simulink model "testsystem2proj"  (R2019b)
settings: Solver=ode23tb  StartTime=0.0  StopTime=0.02  RelTol=1e-3  AbsTol=1e-6
values from neighbouring files (symbols this model uses):
  n = abs(fix(dif/360))    [DE_12.m]
undefined symbols (not defined in the file or in its folder): b, den, dx, flagc, m, minx, num
libraries: powerlib x43, elements x21, simulink_extras x9, powerlib_extras x1
(part 1 of 2)
settings Model: ExtModeTrigMode=oneshot  ExtModeArmWhenConnect=off  Creator=PC  LastModifiedBy=jrooaa06
settings SolverCC: AutoScaleAbsTol=off
settings DataIOCC: SaveFormat=Array  SignalLoggingSaveFormat=ModelDataLogs  ReturnWorkspaceOutputs=off
settings OptimizationCC: BlockReduction=off  BooleanDataType=off  LifeSpan=inf
settings DebuggingCC: SaveWithParameterizedLinksMsg=none  UnderspecifiedInitializationDetection=Classic  MergeDetectMultiDrivingBlocksExec=none  SignalResolutionControl=TryResolveAllWithWarning  MultiTaskDSMMsg=warning  MultiTaskCondExecSysMsg=none  SFUnexpectedBacktrackingDiag=warning  SFNoUnconditionalDefaultTransitionDiag=warning  SFExecutionAtInitializationDiag=none  ArithmeticOperatorsInVariantConditions=warning
settings HardwareCC: ProdBitPerPointer=32  ProdBitPerSizeT=32  ProdBitPerPtrDiffT=32  ProdLargestAtomicFloat=None  ProdIntDivRoundTo=Undefined  ProdEndianess=Unspecified  ProdWordSize=32  ProdHWDeviceType=32-bit Generic  TargetUnknown=on
settings ModelReferenceCC: PropagateSignalLabelsOutOfModel=off
settings SFSimCC: SimUseLocalCustomCode=off  CustomCodeUndefinedFunction=UseInterfaceOnly
settings RTWCC: RTWUseLocalCustomCode=off
settings CodeAppCC: StateflowObjectComments=on
settings GRTTargetCC: TargetLangStandard=C89/C90 (ANSI)  GeneratePreprocessorConditionals=Disable all  CombineOutputUpdateFcns=off  GRTInterface=on
settings ConfigComp: CovMetricSettings=dw  CovHtmlReporting=on  CovSaveCumulativeToWorkspaceVar=on  CovSaveSingleToWorkspaceVar=on  CovExternalEMLEnable=off
settings SimscapeCC: SimscapeNormalizeSystem=off

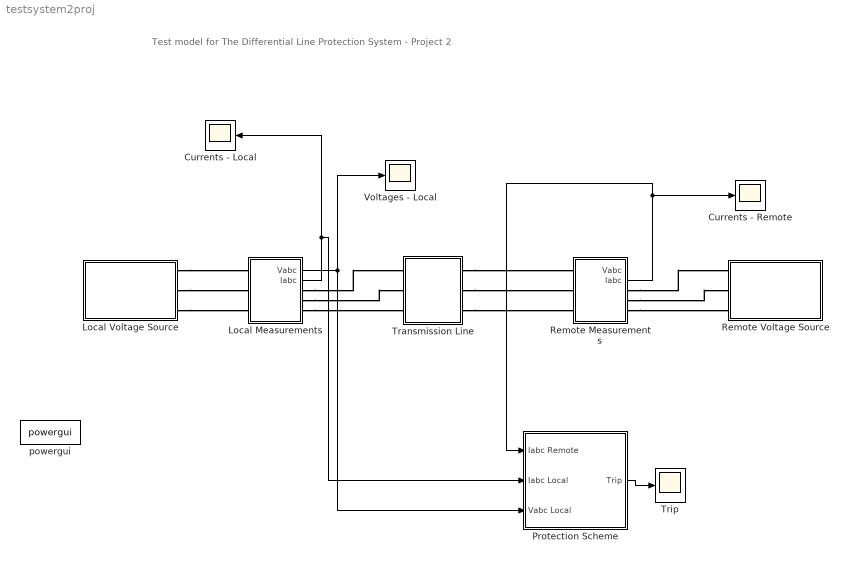
== system testsystem2proj ==
  note: Test model for The Differential Line Protection System - Project 2
  Currents - Local : Scope
  Currents - Remote : Scope
  Local Measurements : Subsystem  mask{VT=2000, CT=100}
      mask prompts: VT "VT ratio"; CT "CT ratio"
  Local Voltage Source : Subsystem  mask(3-phase inductive source - Ungrounded neutral){V=194367, Phi=10, F=60, R=3.4878, L=0.1323}
      mask prompts: V "Voltage magnitude (V) :"; Phi "Phase angle of phase A (Degrees) :"; F "Frequency (Hz) :"; R "Source resistance (Ohms):"; L "Source inductance (H) :"
      mask init:
      | a=R;b=L;c=inf;
      | short_x =[0,150];
      | short_y =[0,0];
      | 
      | resistor_x = [0 30,30,38,53,68,83,98,113,120,120,150];
      | resistor_y = [0,0,0,25,-25,25,-25,25,-25,0,0,0];
      | 
      | inductor_x = [150,173,173,174,178,184,190,197,202,205,206,204,201,201,197,196,198,201,207,214,220,225,229,229,227,224,224,220,219,221,225,230,237,243,249,252,253,251,247,247,244,243,244,248,254,260,267,272,275,276,276,300];
      | 
      | inductor_y = [0,0,1,11,19,24,25,23,17,8,-2,-12,-18,-18,-9,1,11,19,24,25,23,17,8,-2,-12,-18,-18,-9,1,11,19,24,25,23,17,8,-2,-12,-18,-18,-9,1, 11,19,24,25,23,17,8,0,0,0];
      | 
      | capacitor_x1 = [300 360 360 360];
      | capacitor_y1 = [0 0 25 -25];
      | capacitor_x2 = [390 390 390 450];
      | capacitor_y2 = [25,-25,0,0];
      | if a~=0
      | 	s1=resistor_x;
      | 	s2=resistor_y;
      | else
      | 	s1=short_x;
      | 	s2=short_y;
      | end
      | 
      | if b~=0
      | 	s3=inductor_x;
      | 	s4=inductor_y;
      | else
      | 	s3=short_x+150;
      | 	s4=short_y;
      | end
      | 
      | s5=[];
      | s6=[];
      | s7=[];
      | s8=[];
      mask Display: plot(-170,-60,360,60,s1,s2,s3,s4,s5,s6,s7,s8, [0,9,18,24,29,30,29,24,18,9,0,-9,-18,-24,-29,-30,-29,-24,-18,-9,0]*1.5-45,  [30,29,24,18,9,0,-9,-18,-24,-29,-30,-29,-24,-18,-9,0,9,18,24,29,30]*0.8,[-150,-90],[0,0],[-150,-150],[-20,20],[-165,-165],[-15,15],[-180,-180],[-10,10])
  Protection Scheme : Subsystem  mask{bias=[ 0 0;1 0.5 ;3 0.8; 5 4; 7 4.2 ; 8 4.22], Cpg=1e-6, Cpp=1e-7, zone1=[0 0 ;1 0; 1 1; 0.5 1], zone2=[0 0; 2 0; 2 2; 0 2], zone3=[0 0; 3 0; 3 3 ;0 3], zone4=[0 0; 4 0; 5 4; 1 5], reversezone=[0 0; -1 0; -1 -1; 0 -1], delay=[0.001 0.002 0.003 0.001]}
      mask prompts: bias "Bias Characteristic"; Cpg "Capacitance between phase and ground (F)"; Cpp "Mutual Capacitance between phases (F)"; zone1 "Back-up protection zone 1:"; zone2 "Back-up protection zone 2"; zone3 "Back-up protection zone 3"; zone4 "Back-up protection zone 4"; reversezone "Back-up protection reverse zone"; delay "Delay times for zone protection [Z2 Z3 Z4 Reverse]"
  Remote Measurements : Subsystem  mask{VT=2000, CT=100}
      mask prompts: VT "VT ratio"; CT "CT ratio"
  "Remote Voltage Source " : Subsystem  mask(3-phase inductive source - Ungrounded neutral){V=194367, Phi=0, F=60, R=3.4878, L=0.1323}
      mask prompts: V "Voltage magnitude (V) :"; Phi "Phase angle of phase A (Degrees) :"; F "Frequency (Hz) :"; R "Source resistance (Ohms):"; L "Source inductance (H) :"
      mask init: same as testsystem2proj/Local Voltage Source
      mask Display: plot(-170,-60,360,60,s1,s2,s3,s4,s5,s6,s7,s8, [0,9,18,24,29,30,29,24,18,9,0,-9,-18,-24,-29,-30,-29,-24,-18,-9,0]*1.5-45,  [30,29,24,18,9,0,-9,-18,-24,-29,-30,-29,-24,-18,-9,0,9,18,24,29,30]*0.8,[-150,-90],[0,0],[-150,-150],[-20,20],[-165,-165],[-15,15],[-180,-180],[-10,10])
  Transmission Line : Subsystem  mask(Teansmission line with fault){ff=60, rr=[0.0815 0.3666], ll=[2.1e-3 6.5e-3], cc=[31.6e-9 12.7e-9], length=100, faultLocation=0.5, faultType='C-A-G', faultR=0.5, faultTime=[9 10 11 12 13]}
      mask prompts: ff "Frequency used for R L C specification (Hz)"; rr "Resistance per unit length (Ohm/mile) [R1 R0]"; ll "Inductance per unit length (H/mile) [L1 L0]"; cc "Capacitance per unit length (F/mile) [C1 C0]"; length "Line length (mile)"; faultLocation "Fault location (p.u.) <0,1>"; faultType "Fault Type"; faultR "Fault Resistance per Phase (Ohm)"; faultTime "Fault time sequence (s) [C O C O C]"
      mask TypeOptions faultType: 'A-G' | 'B-G' | 'C-G' | 'B-C' | 'B-C-G' | 'C-A' | 'C-A-G' | 'A-B-C' | 'A-B-C-G'
  Trip : Scope
  Voltages - Local : Scope
  powergui : powerlib/powergui  SimulationMode=Continuous  SampleTime=1e-6  frequency=60  Iterations=50  frequencyindice=60  Pbase=100e6  ErrMax=1e-4  UnitsV=kV  UnitsW=MW  buscounter=0  FunctionMessages=off  echomessages=off  EnableUseOfTLC=off  CurrentSourceSwitches=on  DisableSnubberDevices=off  DisableRonSwitches=off  DisableVfSwitches=off  DisplayEquations=off  AutomaticDiscreteSolvers=off  SolverType=Tustin/Backward Euler (TBE)  Interpol=off  ExternalGateDelay=off  methode=off  Ts=0  x0status=blocks  SPID=off  SwTol=0  HookPort=off  NonlinearTolerance=1e-4  nMaxIteration=100  ContinueOnMaxIteration=off  RestoreLinks=warning  ResistiveCurrentMeasurement=off  Frange=[0:2:500]  Ylog=off  Xlog=on  ShowGrid=off  save=off  variable=ZData  structure=0  ZoomFFT=on  StartTime=0.0  cycles=1  DisplayStyle=1  fundamental=60  FreqAxis=off  MaxFrequency=1000  frequencyindicesteady=1  RmsSteady=1  display=off
      settings: SourceProductName=Simscape Electrical
  wires:
  Local Measurements/1(Vabc) -> Voltages - Local/1, Protection Scheme/3(Vabc Local)
  Remote Measurements/2(Iabc) -> Protection Scheme/1(Iabc Remote), Currents - Remote/1
  Protection Scheme/1(Trip) -> Trip/1
  Local Measurements/2(Iabc) -> Protection Scheme/2(Iabc Local), Currents - Local/1
  connections:
  Local Voltage Source/RConn1 -- Local Measurements/LConn1
  Local Voltage Source/RConn2 -- Local Measurements/LConn2
  Local Voltage Source/RConn3 -- Local Measurements/LConn3
  Local Measurements/RConn1 -- Transmission Line/LConn1
  Local Measurements/RConn2 -- Transmission Line/LConn2
  Local Measurements/RConn3 -- Transmission Line/LConn3
  Transmission Line/RConn1 -- Remote Measurements/LConn1
  Transmission Line/RConn2 -- Remote Measurements/LConn2
  Transmission Line/RConn3 -- Remote Measurements/LConn3
  Remote Measurements/RConn1 -- "Remote Voltage Source "/RConn1
  Remote Measurements/RConn2 -- "Remote Voltage Source "/RConn2
  Remote Measurements/RConn3 -- "Remote Voltage Source "/RConn3

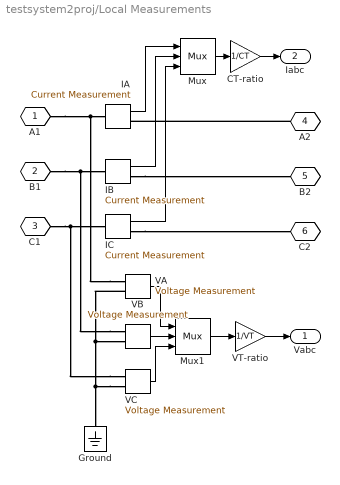
== system testsystem2proj/Local Measurements ==
  CT-ratio : Gain  Gain=1/CT  SaturateOnIntegerOverflow=on  OutDataTypeStr=Inherit: Same as input  ParamDataTypeStr=Inherit: Same as input
  Ground : powerlib/Elements/Ground  LConnTagsString=a
      settings: SourceProductName=Simscape Electrical
  IA : powerlib/Measurements/Current Measurement  PhasorSimulation=off  OutputType=Complex  PSBequivalent=0
      settings: SourceProductName=Simscape Electrical
  IB : powerlib/Measurements/Current Measurement  PhasorSimulation=off  OutputType=Complex  PSBequivalent=0
      settings: SourceProductName=Simscape Electrical
  IC : powerlib/Measurements/Current Measurement  PhasorSimulation=off  OutputType=Complex  PSBequivalent=0
      settings: SourceProductName=Simscape Electrical
  Mux : Mux  Inputs=3
  Mux1 : Mux  Inputs=3
  VA : powerlib/Measurements/Voltage Measurement  PhasorSimulation=off  OutputType=Complex  PSBequivalent=0
      settings: SourceProductName=Simscape Electrical
  VB : powerlib/Measurements/Voltage Measurement  PhasorSimulation=off  OutputType=Complex  PSBequivalent=0
      settings: SourceProductName=Simscape Electrical
  VC : powerlib/Measurements/Voltage Measurement  PhasorSimulation=off  OutputType=Complex  PSBequivalent=0
      settings: SourceProductName=Simscape Electrical
  VT-ratio : Gain  Gain=1/VT  SaturateOnIntegerOverflow=on  OutDataTypeStr=Inherit: Same as input  ParamDataTypeStr=Inherit: Same as input
  A1 : PMIOPort  Tag=PMCPort  Side=Left
  B1 : PMIOPort  Tag=PMCPort  Port=2  Side=Left
  C1 : PMIOPort  Tag=PMCPort  Port=3  Side=Left
  A2 : PMIOPort  Tag=PMCPort  Port=4  Side=Right
  B2 : PMIOPort  Tag=PMCPort  Port=5  Side=Right
  C2 : PMIOPort  Tag=PMCPort  Port=6  Side=Right
  Vabc : Outport  InitialOutput=0
  Iabc : Outport  Port=2  InitialOutput=0
  wires:
  VC/1 -> Mux1/3
  VB/1 -> Mux1/2
  VA/1 -> Mux1/1
  CT-ratio/1 -> Iabc/1
  Mux/1 -> CT-ratio/1
  VT-ratio/1 -> Vabc/1
  Mux1/1 -> VT-ratio/1
  IA/1 -> Mux/1
  IB/1 -> Mux/2
  IC/1 -> Mux/3
  connections:
  IC/RConn1 -- C2/RConn1
  IB/RConn1 -- B2/RConn1
  A2/RConn1 -- IA/RConn1
  VC/LConn1 -- IC/LConn1 -- C1/RConn1
  VB/LConn1 -- IB/LConn1 -- B1/RConn1
  VA/LConn1 -- IA/LConn1 -- A1/RConn1
  VC/LConn2 -- Ground/LConn1 -- VB/LConn2 -- VA/LConn2

== system testsystem2proj/Local Voltage Source ==
  Ground : powerlib/Elements/Ground  LConnTagsString=a
      settings: SourceProductName=Simscape Electrical
  RA : powerlib/Elements/Series RLC Branch  LConnTagsString=__new0  RConnTagsString=__new0  BranchType=RL  Resistance=R  Inductance=L  SetiL0=off  InitialCurrent=0  Capacitance=1.0  Setx0=off  InitialVoltage=0  Measurements=None
      settings: SourceProductName=Simscape Electrical
  RB : powerlib/Elements/Series RLC Branch  LConnTagsString=__new0  RConnTagsString=__new0  BranchType=RL  Resistance=R  Inductance=L  SetiL0=off  InitialCurrent=0  Capacitance=1.0  Setx0=off  InitialVoltage=0  Measurements=None
      settings: SourceProductName=Simscape Electrical
  RC : powerlib/Elements/Series RLC Branch  LConnTagsString=__new0  RConnTagsString=__new0  BranchType=RL  Resistance=R  Inductance=L  SetiL0=off  InitialCurrent=0  Capacitance=1.0  Setx0=off  InitialVoltage=0  Measurements=None
      settings: SourceProductName=Simscape Electrical
  VA : powerlib/Electrical Sources/AC Voltage Source  Amplitude=V  Phase=Phi  Frequency=F  SampleTime=0  Measurements=None  BusType=swing  Pref=10e3  Qref=0  Qmin=-inf  Qmax=+inf
      settings: SourceProductName=Simscape Electrical
  VB : powerlib/Electrical Sources/AC Voltage Source  Amplitude=V  Phase=Phi-120  Frequency=F  SampleTime=0  Measurements=None  BusType=swing  Pref=10e3  Qref=0  Qmin=-inf  Qmax=+inf
      settings: SourceProductName=Simscape Electrical
  VC : powerlib/Electrical Sources/AC Voltage Source  Amplitude=V  Phase=Phi+120  Frequency=F  SampleTime=0  Measurements=None  BusType=swing  Pref=10e3  Qref=0  Qmin=-inf  Qmax=+inf
      settings: SourceProductName=Simscape Electrical
  A : PMIOPort  Tag=PMCPort  Side=Right
  B : PMIOPort  Tag=PMCPort  Port=2  Side=Right
  C : PMIOPort  Tag=PMCPort  Port=3  Side=Right
  connections:
  VC/LConn1 -- VA/LConn1 -- Ground/LConn1 -- VB/LConn1
  VA/RConn1 -- RA/LConn1
  VB/RConn1 -- RB/LConn1
  VC/RConn1 -- RC/LConn1
  RA/RConn1 -- A/RConn1
  RB/RConn1 -- B/RConn1
  RC/RConn1 -- C/RConn1

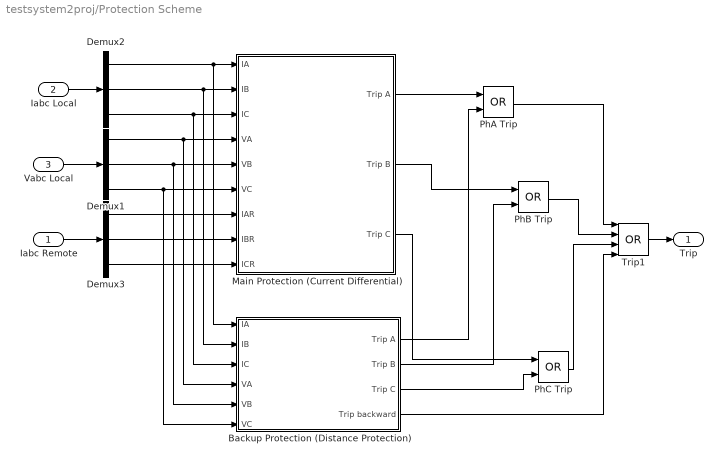
== system testsystem2proj/Protection Scheme ==
  Iabc Remote : Inport
  Iabc Local : Inport  Port=2
  Vabc Local : Inport  Port=3
  Backup Protection (Distance Protection) : Subsystem
  Demux1 : Demux  Outputs=3
  Demux2 : Demux  Outputs=3
  Demux3 : Demux  Outputs=3
  Main Protection (Current Differential) : Subsystem
  PhA Trip : Logic  Operator=OR
  PhB Trip : Logic  Operator=OR
  PhC Trip : Logic  Operator=OR
  Trip1 : Logic  Operator=OR  Inputs=4
  Trip : Outport
  wires:
  Vabc Local/1 -> Demux1/1
  Iabc Local/1 -> Demux2/1
  Iabc Remote/1 -> Demux3/1
  Trip1/1 -> Trip/1
  PhA Trip/1 -> Trip1/1
  PhB Trip/1 -> Trip1/2
  PhC Trip/1 -> Trip1/3
  Backup Protection (Distance Protection)/1(Trip A) -> PhA Trip/2
  Backup Protection (Distance Protection)/2(Trip B) -> PhB Trip/2
  Backup Protection (Distance Protection)/3(Trip C) -> PhC Trip/2
  Demux3/1 -> Main Protection (Current Differential)/7(IAR)
  Demux3/2 -> Main Protection (Current Differential)/8(IBR)
  Demux3/3 -> Main Protection (Current Differential)/9(ICR)
  Demux2/1 -> Main Protection (Current Differential)/1(IA), Backup Protection (Distance Protection)/1(IA)
  Demux2/2 -> Main Protection (Current Differential)/2(IB), Backup Protection (Distance Protection)/2(IB)
  Demux2/3 -> Main Protection (Current Differential)/3(IC), Backup Protection (Distance Protection)/3(IC)
  Demux1/1 -> Main Protection (Current Differential)/4(VA), Backup Protection (Distance Protection)/4(VA)
  Demux1/2 -> Main Protection (Current Differential)/5(VB), Backup Protection (Distance Protection)/5(VB)
  Demux1/3 -> Main Protection (Current Differential)/6(VC), Backup Protection (Distance Protection)/6(VC)
  Backup Protection (Distance Protection)/4(Trip backward) -> Trip1/4
  Main Protection (Current Differential)/1(Trip A) -> PhA Trip/1
  Main Protection (Current Differential)/2(Trip B) -> PhB Trip/1
  Main Protection (Current Differential)/3(Trip C) -> PhC Trip/1

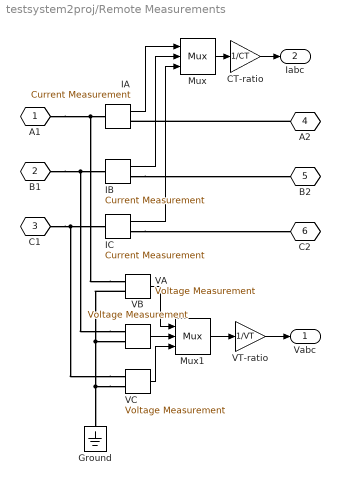
== system testsystem2proj/Remote Measurements ==
  CT-ratio : Gain  Gain=1/CT  SaturateOnIntegerOverflow=on  OutDataTypeStr=Inherit: Same as input  ParamDataTypeStr=Inherit: Same as input
  Ground : powerlib/Elements/Ground  LConnTagsString=a
      settings: SourceProductName=Simscape Electrical
  IA : powerlib/Measurements/Current Measurement  PhasorSimulation=off  OutputType=Complex  PSBequivalent=0
      settings: SourceProductName=Simscape Electrical
  IB : powerlib/Measurements/Current Measurement  PhasorSimulation=off  OutputType=Complex  PSBequivalent=0
      settings: SourceProductName=Simscape Electrical
  IC : powerlib/Measurements/Current Measurement  PhasorSimulation=off  OutputType=Complex  PSBequivalent=0
      settings: SourceProductName=Simscape Electrical
  Mux : Mux  Inputs=3
  Mux1 : Mux  Inputs=3
  VA : powerlib/Measurements/Voltage Measurement  PhasorSimulation=off  OutputType=Complex  PSBequivalent=0
      settings: SourceProductName=Simscape Electrical
  VB : powerlib/Measurements/Voltage Measurement  PhasorSimulation=off  OutputType=Complex  PSBequivalent=0
      settings: SourceProductName=Simscape Electrical
  VC : powerlib/Measurements/Voltage Measurement  PhasorSimulation=off  OutputType=Complex  PSBequivalent=0
      settings: SourceProductName=Simscape Electrical
  VT-ratio : Gain  Gain=1/VT  SaturateOnIntegerOverflow=on  OutDataTypeStr=Inherit: Same as input  ParamDataTypeStr=Inherit: Same as input
  A1 : PMIOPort  Tag=PMCPort  Side=Left
  B1 : PMIOPort  Tag=PMCPort  Port=2  Side=Left
  C1 : PMIOPort  Tag=PMCPort  Port=3  Side=Left
  A2 : PMIOPort  Tag=PMCPort  Port=4  Side=Right
  B2 : PMIOPort  Tag=PMCPort  Port=5  Side=Right
  C2 : PMIOPort  Tag=PMCPort  Port=6  Side=Right
  Vabc : Outport  InitialOutput=0
  Iabc : Outport  Port=2  InitialOutput=0
  wires:
  VC/1 -> Mux1/3
  VB/1 -> Mux1/2
  VA/1 -> Mux1/1
  CT-ratio/1 -> Iabc/1
  Mux/1 -> CT-ratio/1
  VT-ratio/1 -> Vabc/1
  Mux1/1 -> VT-ratio/1
  IA/1 -> Mux/1
  IB/1 -> Mux/2
  IC/1 -> Mux/3
  connections:
  IC/RConn1 -- C2/RConn1
  IB/RConn1 -- B2/RConn1
  A2/RConn1 -- IA/RConn1
  VC/LConn1 -- IC/LConn1 -- C1/RConn1
  VB/LConn1 -- IB/LConn1 -- B1/RConn1
  VA/LConn1 -- IA/LConn1 -- A1/RConn1
  VC/LConn2 -- Ground/LConn1 -- VB/LConn2 -- VA/LConn2

== system testsystem2proj/Remote Voltage Source  ==
  Ground : powerlib/Elements/Ground  LConnTagsString=a
      settings: SourceProductName=Simscape Electrical
  RA : powerlib/Elements/Series RLC Branch  LConnTagsString=__new0  RConnTagsString=__new0  BranchType=RL  Resistance=R  Inductance=L  SetiL0=off  InitialCurrent=0  Capacitance=1.0  Setx0=off  InitialVoltage=0  Measurements=None
      settings: SourceProductName=Simscape Electrical
  RB : powerlib/Elements/Series RLC Branch  LConnTagsString=__new0  RConnTagsString=__new0  BranchType=RL  Resistance=R  Inductance=L  SetiL0=off  InitialCurrent=0  Capacitance=1.0  Setx0=off  InitialVoltage=0  Measurements=None
      settings: SourceProductName=Simscape Electrical
  RC : powerlib/Elements/Series RLC Branch  LConnTagsString=__new0  RConnTagsString=__new0  BranchType=RL  Resistance=R  Inductance=L  SetiL0=off  InitialCurrent=0  Capacitance=1.0  Setx0=off  InitialVoltage=0  Measurements=None
      settings: SourceProductName=Simscape Electrical
  VA : powerlib/Electrical Sources/AC Voltage Source  Amplitude=V  Phase=Phi  Frequency=F  SampleTime=0  Measurements=Voltage  BusType=swing  Pref=10e3  Qref=0  Qmin=-inf  Qmax=+inf
      settings: SourceProductName=Simscape Electrical
  VB : powerlib/Electrical Sources/AC Voltage Source  Amplitude=V  Phase=Phi-120  Frequency=F  SampleTime=0  Measurements=Voltage  BusType=swing  Pref=10e3  Qref=0  Qmin=-inf  Qmax=+inf
      settings: SourceProductName=Simscape Electrical
  VC : powerlib/Electrical Sources/AC Voltage Source  Amplitude=V  Phase=Phi+120  Frequency=F  SampleTime=0  Measurements=None  BusType=swing  Pref=10e3  Qref=0  Qmin=-inf  Qmax=+inf
      settings: SourceProductName=Simscape Electrical
  A : PMIOPort  Tag=PMCPort  Side=Right
  B : PMIOPort  Tag=PMCPort  Port=2  Side=Right
  C : PMIOPort  Tag=PMCPort  Port=3  Side=Right
  connections:
  RC/RConn1 -- C/RConn1
  RB/RConn1 -- B/RConn1
  RA/RConn1 -- A/RConn1
  VC/RConn1 -- RC/LConn1
  VB/RConn1 -- RB/LConn1
  VA/RConn1 -- RA/LConn1
  VB/LConn1 -- Ground/LConn1 -- VA/LConn1 -- VC/LConn1

== system testsystem2proj/Transmission Line ==
  Fault : Subsystem
  Fault Selector : Subsystem
  Line1 : powerlib/Elements/Distributed Parameters Line  Phases=3  Frequency=ff  Resistance=rr  Inductance=ll  Capacitance=cc  Length=length*faultLocation  x1=[1.93737315649841e-10 244713.938533905 244713.938533905;376.991118430775 376.991118430775 376.991118430775;-1.14363890113431 0.490220023006083 -1.08057630378881]  x2=[4.17528404371218e-10 247270.406287336 247270.406287336;376.991118430775 376.991118430775 376.991118430775;-0.895009460576135 0.449233113533289 -1.12156321326161]  x3=[2.62101290427986e-12 709.319312320514 709.319312320518;376.991118430775 376.991118430775 376.991118430775;-2.01300464495126 0.267353068449138 -1.30344325834575]  x4=[1.05439609711696e-12 1190.69642129133 1190.69642129132;376.991118430775 376.991118430775 376.991118430775;0.959692276161214 0.466990655381244 -1.10380567141365]  x5=0.000454285152739994  V1=[1.937e-10 2.447e+05 2.447e+05;377 377 377;-1.144 0.4902 -1.081]  V2=[4.175e-10 2.473e+05 2.473e+05;377 377 377;-0.895 0.4492 -1.122]  I1=[2.621e-12 709.3 709.3;377 377 377;-2.013 0.2674 -1.303]  I2=[1.054e-12 1191 1191;377 377 377;0.9597 0.467 -1.104]  nHarmo=1  Measurements=None
      settings: SourceProductName=Simscape Electrical
  Line2 : powerlib/Elements/Distributed Parameters Line  Phases=3  Frequency=ff  Resistance=rr  Inductance=ll  Capacitance=cc  Length=length*(1-faultLocation)  x1=[4.17528404371218e-10 247270.406287336 247270.406287336;376.991118430775 376.991118430775 376.991118430775;-0.895009460576135 0.449233113533289 -1.12156321326161]  x2=[2.82547085064981e-10 244460.357066528 244460.357066528;376.991118430775 376.991118430775 376.991118430775;-0.77354881395291 0.41468188233202 -1.15611444446288]  x3=[6.1795565465611e-13 730.365390861983 730.365390861978;376.991118430775 376.991118430775 376.991118430775;-0.860185856032807 0.42028091422424 -1.15051541257066]  x4=[1.68453032078769e-12 1162.47547836006 1162.47547836006;376.991118430775 376.991118430775 376.991118430775;-2.26533611674482 0.313964295998751 -1.25683203079614]  x5=0.000454285152739994  V1=[4.175e-10 2.473e+05 2.473e+05;377 377 377;-0.895 0.4492 -1.122]  V2=[2.825e-10 2.445e+05 2.445e+05;377 377 377;-0.7735 0.4147 -1.156]  I1=[6.18e-13 730.4 730.4;377 377 377;-0.8602 0.4203 -1.151]  I2=[1.685e-12 1162 1162;377 377 377;-2.265 0.314 -1.257]  nHarmo=1  Measurements=None
      settings: SourceProductName=Simscape Electrical
  Timer : powerlib_extras/Control  Blocks/Timer  t=[0 faultTime]  e=[0 1 0 1 0 1]
      settings: SourceProductName=Simscape Electrical  SourceProductBaseCode=PS
  A1 : PMIOPort  Tag=PMCPort  Side=Left
  B1 : PMIOPort  Tag=PMCPort  Port=2  Side=Left
  C1 : PMIOPort  Tag=PMCPort  Port=3  Side=Left
  A2 : PMIOPort  Tag=PMCPort  Port=4  Side=Right
  B2 : PMIOPort  Tag=PMCPort  Port=5  Side=Right
  C2 : PMIOPort  Tag=PMCPort  Port=6  Side=Right
  wires:
  Timer/1 -> Fault/5(Tfault)
  Fault Selector/4(faultG) -> Fault/4(faultG)
  Fault Selector/3(faultC) -> Fault/3(faultC)
  Fault Selector/2(faultB) -> Fault/2(faultB)
  Fault Selector/1(faultA) -> Fault/1(faultA)
  connections:
  Line2/RConn3 -- C2/RConn1
  Line2/RConn2 -- B2/RConn1
  Line2/RConn1 -- A2/RConn1
  C1/RConn1 -- Line1/LConn3
  B1/RConn1 -- Line1/LConn2
  A1/RConn1 -- Line1/LConn1
  Fault/LConn3 -- Line1/RConn3 -- Line2/LConn3
  Fault/LConn2 -- Line2/LConn2 -- Line1/RConn2
  Fault/LConn1 -- Line2/LConn1 -- Line1/RConn1

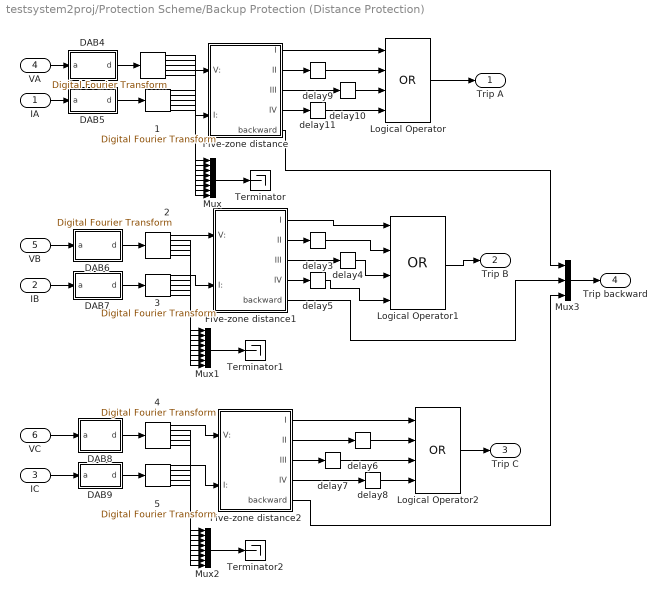
== system testsystem2proj/Protection Scheme/Backup Protection (Distance Protection) ==
  IA : Inport
  IB : Inport  Port=2
  IC : Inport  Port=3
  VA : Inport  Port=4
  VB : Inport  Port=5
  VC : Inport  Port=6
   {,1..5} (6 alike) : elements/   fo=60  window_size=40  harmonic=[1 2 3 4 5]
  DAB4 : Subsystem  mask(Data Adquisition Board){filter=off, approx=Bessel, order=2, numerator=[], denominator=[], freq=180, resdis=off, vertres=12, xmax=10, winsize=40, G=1.0, fs=60*40}
      mask prompts: filter "Disable Analog Filter"; approx "Filter approximation"; numerator "Free expression filter: numerator(descending order of s)"; denominator "Free expression filter: denominator:"; freq "Cut-off frequency"; resdis "Disable Vertical Resolution"; vertres "Vertical Resolution: No. of bits"; xmax "Vertical Resolution: signal range"; winsize "Window size"; G "Gain"; fs "Sampling frequency"
      mask help: Performs analog filtering, signal conditioning and sampling. A single signal is the input, a buffer with the signal samples is the output. The options include analog filter enable/disable switch, type, order and cut-off frequency of the analog filter, conditioning gain, sampling frequency, number of bits, the length of the buffer.
      mask init:
      | dab1
      mask TypeOptions approx: Bessel | Tschebyscheff | Butterworth | free expression
      mask TypeOptions order: 2 | 3 | 4
      mask TypeOptions vertres: 8 | 12 | 16
      mask Display: disp('DAB')
  DAB5 : Subsystem  mask(Data Adquisition Board){filter=off, approx=Bessel, order=2, numerator=[], denominator=[], freq=180, resdis=off, vertres=12, xmax=10, winsize=40, G=1.0, fs=60*40}
      mask prompts: filter "Disable Analog Filter"; approx "Filter approximation"; numerator "Free expression filter: numerator(descending order of s)"; denominator "Free expression filter: denominator:"; freq "Cut-off frequency"; resdis "Disable Vertical Resolution"; vertres "Vertical Resolution: No. of bits"; xmax "Vertical Resolution: signal range"; winsize "Window size"; G "Gain"; fs "Sampling frequency"
      mask help: Performs analog filtering, signal conditioning and sampling. A single signal is the input, a buffer with the signal samples is the output. The options include analog filter enable/disable switch, type, order and cut-off frequency of the analog filter, conditioning gain, sampling frequency, number of bits, the length of the buffer.
      mask init:
      | dab1
      mask TypeOptions approx: Bessel | Tschebyscheff | Butterworth | free expression
      mask TypeOptions order: 2 | 3 | 4
      mask TypeOptions vertres: 8 | 12 | 16
      mask Display: disp('DAB')
  DAB6 : Subsystem  mask(Data Adquisition Board){filter=off, approx=Bessel, order=2, numerator=[], denominator=[], freq=180, resdis=off, vertres=12, xmax=10, winsize=40, G=1.0, fs=60*40}
      mask prompts: filter "Disable Analog Filter"; approx "Filter approximation"; numerator "Free expression filter: numerator(descending order of s)"; denominator "Free expression filter: denominator:"; freq "Cut-off frequency"; resdis "Disable Vertical Resolution"; vertres "Vertical Resolution: No. of bits"; xmax "Vertical Resolution: signal range"; winsize "Window size"; G "Gain"; fs "Sampling frequency"
      mask help: Performs analog filtering, signal conditioning and sampling. A single signal is the input, a buffer with the signal samples is the output. The options include analog filter enable/disable switch, type, order and cut-off frequency of the analog filter, conditioning gain, sampling frequency, number of bits, the length of the buffer.
      mask init:
      | dab1
      mask TypeOptions approx: Bessel | Tschebyscheff | Butterworth | free expression
      mask TypeOptions order: 2 | 3 | 4
      mask TypeOptions vertres: 8 | 12 | 16
      mask Display: disp('DAB')
  DAB7 : Subsystem  mask(Data Adquisition Board){filter=off, approx=Bessel, order=2, numerator=[], denominator=[], freq=180, resdis=off, vertres=12, xmax=10, winsize=40, G=1.0, fs=60*40}
      mask prompts: filter "Disable Analog Filter"; approx "Filter approximation"; numerator "Free expression filter: numerator(descending order of s)"; denominator "Free expression filter: denominator:"; freq "Cut-off frequency"; resdis "Disable Vertical Resolution"; vertres "Vertical Resolution: No. of bits"; xmax "Vertical Resolution: signal range"; winsize "Window size"; G "Gain"; fs "Sampling frequency"
      mask help: Performs analog filtering, signal conditioning and sampling. A single signal is the input, a buffer with the signal samples is the output. The options include analog filter enable/disable switch, type, order and cut-off frequency of the analog filter, conditioning gain, sampling frequency, number of bits, the length of the buffer.
      mask init:
      | dab1
      mask TypeOptions approx: Bessel | Tschebyscheff | Butterworth | free expression
      mask TypeOptions order: 2 | 3 | 4
      mask TypeOptions vertres: 8 | 12 | 16
      mask Display: disp('DAB')
  DAB8 : Subsystem  mask(Data Adquisition Board){filter=off, approx=Bessel, order=2, numerator=[], denominator=[], freq=180, resdis=off, vertres=12, xmax=10, winsize=40, G=1.0, fs=60*40}
      mask prompts: filter "Disable Analog Filter"; approx "Filter approximation"; numerator "Free expression filter: numerator(descending order of s)"; denominator "Free expression filter: denominator:"; freq "Cut-off frequency"; resdis "Disable Vertical Resolution"; vertres "Vertical Resolution: No. of bits"; xmax "Vertical Resolution: signal range"; winsize "Window size"; G "Gain"; fs "Sampling frequency"
      mask help: Performs analog filtering, signal conditioning and sampling. A single signal is the input, a buffer with the signal samples is the output. The options include analog filter enable/disable switch, type, order and cut-off frequency of the analog filter, conditioning gain, sampling frequency, number of bits, the length of the buffer.
      mask init:
      | dab1
      mask TypeOptions approx: Bessel | Tschebyscheff | Butterworth | free expression
      mask TypeOptions order: 2 | 3 | 4
      mask TypeOptions vertres: 8 | 12 | 16
      mask Display: disp('DAB')
  DAB9 : Subsystem  mask(Data Adquisition Board){filter=off, approx=Bessel, order=2, numerator=[], denominator=[], freq=180, resdis=off, vertres=12, xmax=10, winsize=40, G=1.0, fs=60*40}
      mask prompts: filter "Disable Analog Filter"; approx "Filter approximation"; numerator "Free expression filter: numerator(descending order of s)"; denominator "Free expression filter: denominator:"; freq "Cut-off frequency"; resdis "Disable Vertical Resolution"; vertres "Vertical Resolution: No. of bits"; xmax "Vertical Resolution: signal range"; winsize "Window size"; G "Gain"; fs "Sampling frequency"
      mask help: Performs analog filtering, signal conditioning and sampling. A single signal is the input, a buffer with the signal samples is the output. The options include analog filter enable/disable switch, type, order and cut-off frequency of the analog filter, conditioning gain, sampling frequency, number of bits, the length of the buffer.
      mask init:
      | dab1
      mask TypeOptions approx: Bessel | Tschebyscheff | Butterworth | free expression
      mask TypeOptions order: 2 | 3 | 4
      mask TypeOptions vertres: 8 | 12 | 16
      mask Display: disp('DAB')
  Five-zone distance : Subsystem
  Five-zone distance1 : Subsystem
  Five-zone distance2 : Subsystem
  Logical Operator : Logic  Operator=OR  Inputs=4
  Logical Operator1 : Logic  Operator=OR  Inputs=4
  Logical Operator2 : Logic  Operator=OR  Inputs=4
  Mux : Mux  Inputs=8
  Mux1 : Mux  Inputs=8
  Mux2 : Mux  Inputs=8
  Mux3 : Mux  Inputs=3
  Terminator : Terminator
  Terminator1 : Terminator
  Terminator2 : Terminator
  delay10 : TransportDelay  DelayTime=delay(2)
  delay11 : TransportDelay  DelayTime=delay(3)
  delay3 : TransportDelay  DelayTime=delay(1)
  delay4 : TransportDelay  DelayTime=delay(2)
  delay5 : TransportDelay  DelayTime=delay(3)
  delay6 : TransportDelay  DelayTime=delay(1)
  delay7 : TransportDelay  DelayTime=delay(2)
  delay8 : TransportDelay  DelayTime=delay(3)
  delay9 : TransportDelay  DelayTime=delay(1)
  Trip A : Outport
  Trip B : Outport  Port=2
  Trip C : Outport  Port=3
  Trip backward : Outport  Port=4
  wires:
  Five-zone distance1/1(I) -> Logical Operator1/1
  " 4"/1 -> Five-zone distance2/1(V:)
  DAB9/1(d) -> " 5"/1
  DAB8/1(d) -> " 4"/1
  VC/1 -> DAB8/1(a)
  IC/1 -> DAB9/1(a)
  Logical Operator2/1 -> Trip C/1
  " 2"/1 -> Five-zone distance1/1(V:)
  DAB7/1(d) -> " 3"/1
  DAB6/1(d) -> " 2"/1
  " 3"/1 -> Five-zone distance1/2(I:)
  Five-zone distance1/2(II) -> delay3/1
  Five-zone distance1/3(III) -> delay4/1
  Five-zone distance1/4(IV) -> delay5/1
  delay3/1 -> Logical Operator1/2
  delay4/1 -> Logical Operator1/3
  delay5/1 -> Logical Operator1/4
  VB/1 -> DAB6/1(a)
  IB/1 -> DAB7/1(a)
  Logical Operator1/1 -> Trip B/1
  " "/1 -> Five-zone distance/1(V:)
  DAB5/1(d) -> " 1"/1
  DAB4/1(d) -> " "/1
  " 1"/1 -> Five-zone distance/2(I:)
  Five-zone distance/1(I) -> Logical Operator/1
  VA/1 -> DAB4/1(a)
  IA/1 -> DAB5/1(a)
  Logical Operator/1 -> Trip A/1
  " "/3 -> Mux/1
  " "/2 -> Mux/2
  " "/4 -> Mux/3
  " "/5 -> Mux/4
  " 1"/2 -> Mux/5
  " 1"/3 -> Mux/6
  " 1"/4 -> Mux/7
  " 1"/5 -> Mux/8
  " 2"/2 -> Mux1/1
  " 2"/3 -> Mux1/2
  " 2"/4 -> Mux1/3
  " 2"/5 -> Mux1/4
  " 3"/2 -> Mux1/5
  " 3"/3 -> Mux1/6
  " 3"/4 -> Mux1/7
  " 3"/5 -> Mux1/8
  " 4"/3 -> Mux2/1
  " 4"/2 -> Mux2/2
  " 4"/4 -> Mux2/3
  " 4"/5 -> Mux2/4
  " 5"/2 -> Mux2/5
  " 5"/3 -> Mux2/6
  " 5"/4 -> Mux2/7
  " 5"/5 -> Mux2/8
  Five-zone distance/5(backward) -> Mux3/1
  Five-zone distance1/5(backward) -> Mux3/2
  " 5"/1 -> Five-zone distance2/2(I:)
  delay6/1 -> Logical Operator2/2
  delay7/1 -> Logical Operator2/3
  delay8/1 -> Logical Operator2/4
  Five-zone distance2/1(I) -> Logical Operator2/1
  Five-zone distance2/2(II) -> delay6/1
  Five-zone distance2/3(III) -> delay7/1
  Five-zone distance2/4(IV) -> delay8/1
  Five-zone distance2/5(backward) -> Mux3/3
  Five-zone distance/2(II) -> delay9/1
  delay9/1 -> Logical Operator/2
  Five-zone distance/3(III) -> delay10/1
  Five-zone distance/4(IV) -> delay11/1
  Mux/1 -> Terminator/1
  Mux1/1 -> Terminator1/1
  Mux2/1 -> Terminator2/1
  delay10/1 -> Logical Operator/3
  delay11/1 -> Logical Operator/4
  Mux3/1 -> Trip backward/1

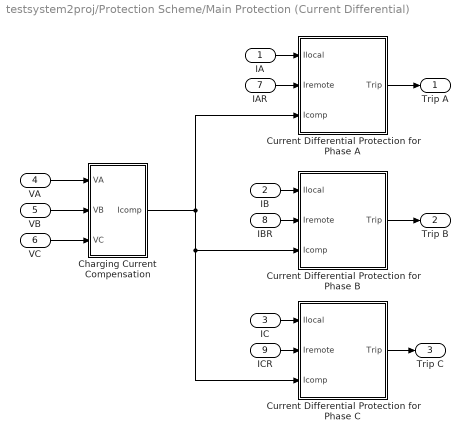
== system testsystem2proj/Protection Scheme/Main Protection (Current Differential) ==
  IA : Inport
  IB : Inport  Port=2
  IC : Inport  Port=3
  VA : Inport  Port=4
  VB : Inport  Port=5
  VC : Inport  Port=6
  IAR : Inport  Port=7
  IBR : Inport  Port=8
  ICR : Inport  Port=9
  Charging Current Compensation : Subsystem
  Current Differential Protection for Phase A : Subsystem
  Current Differential Protection for Phase B : Subsystem
  Current Differential Protection for Phase C : Subsystem
  Trip A : Outport  InitialOutput=0
  Trip B : Outport  Port=2  InitialOutput=0
  Trip C : Outport  Port=3  InitialOutput=0
  wires:
  IA/1 -> Current Differential Protection for Phase A/1(Ilocal)
  IAR/1 -> Current Differential Protection for Phase A/2(Iremote)
  IB/1 -> Current Differential Protection for Phase B/1(Ilocal)
  Current Differential Protection for Phase C/1(Trip) -> Trip C/1
  Current Differential Protection for Phase A/1(Trip) -> Trip A/1
  Current Differential Protection for Phase B/1(Trip) -> Trip B/1
  VB/1 -> Charging Current Compensation/2(VB)
  IBR/1 -> Current Differential Protection for Phase B/2(Iremote)
  IC/1 -> Current Differential Protection for Phase C/1(Ilocal)
  VA/1 -> Charging Current Compensation/1(VA)
  VC/1 -> Charging Current Compensation/3(VC)
  ICR/1 -> Current Differential Protection for Phase C/2(Iremote)
  Charging Current Compensation/1(Icomp) -> Current Differential Protection for Phase A/3(Icomp), Current Differential Protection for Phase B/3(Icomp), Current Differential Protection for Phase C/3(Icomp)

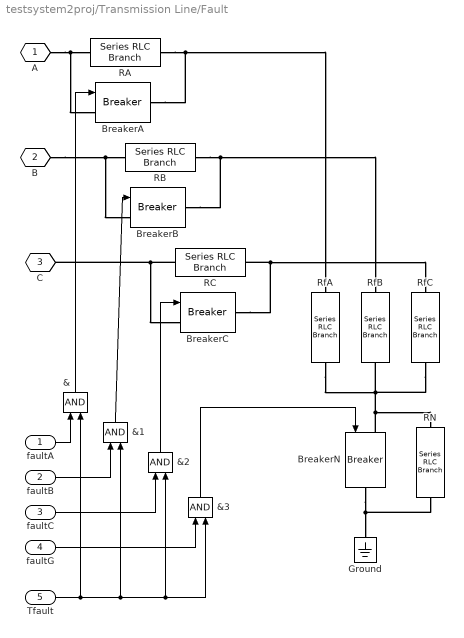
== system testsystem2proj/Transmission Line/Fault ==
  faultA : Inport
  faultB : Inport  Port=2
  faultC : Inport  Port=3
  faultG : Inport  Port=4
  Tfault : Inport  Port=5
  &{,1..3} (4 alike) : Logic
  BreakerA : powerlib/Elements/Breaker  InitialState=0  SwitchingTimes="[ 1/60  5/60 ]"  External=on  BreakerResistance=0.01  SnubberResistance=1e6  SnubberCapacitance=inf  Measurements=None  MoreParameters=off  NoBreakLoop=off
      settings: SourceProductName=Simscape Electrical
  BreakerB : powerlib/Elements/Breaker  InitialState=0  SwitchingTimes="[ 1/60  5/60 ]"  External=on  BreakerResistance=0.01  SnubberResistance=1e6  SnubberCapacitance=inf  Measurements=None  MoreParameters=off  NoBreakLoop=off
      settings: SourceProductName=Simscape Electrical
  BreakerC : powerlib/Elements/Breaker  InitialState=0  SwitchingTimes="[ 1/60  5/60 ]"  External=on  BreakerResistance=0.01  SnubberResistance=1e6  SnubberCapacitance=inf  Measurements=None  MoreParameters=off  NoBreakLoop=off
      settings: SourceProductName=Simscape Electrical
  BreakerN : powerlib/Elements/Breaker  InitialState=0  SwitchingTimes="[ 1/60  5/60 ]"  External=on  BreakerResistance=0.01  SnubberResistance=1e6  SnubberCapacitance=inf  Measurements=None  MoreParameters=off  NoBreakLoop=off
      settings: SourceProductName=Simscape Electrical
  Ground : powerlib/Elements/Ground  LConnTagsString=a
      settings: SourceProductName=Simscape Electrical
  RA : powerlib/Elements/Series RLC Branch  LConnTagsString=__new0  RConnTagsString=__new0  BranchType=R  Resistance=10000  Inductance=1e-3  SetiL0=off  InitialCurrent=0  Capacitance=1e-6  Setx0=off  InitialVoltage=0  Measurements=None
      settings: SourceProductName=Simscape Electrical
  RB : powerlib/Elements/Series RLC Branch  LConnTagsString=__new0  RConnTagsString=__new0  BranchType=R  Resistance=10000  Inductance=1e-3  SetiL0=off  InitialCurrent=0  Capacitance=1e-6  Setx0=off  InitialVoltage=0  Measurements=None
      settings: SourceProductName=Simscape Electrical
  RC : powerlib/Elements/Series RLC Branch  LConnTagsString=__new0  RConnTagsString=__new0  BranchType=R  Resistance=10000  Inductance=1e-3  SetiL0=off  InitialCurrent=0  Capacitance=1e-6  Setx0=off  InitialVoltage=0  Measurements=None
      settings: SourceProductName=Simscape Electrical
  RN : powerlib/Elements/Series RLC Branch  LConnTagsString=__new0  RConnTagsString=__new0  BranchType=R  Resistance=10000  Inductance=1e-3  SetiL0=off  InitialCurrent=0  Capacitance=1e-6  Setx0=off  InitialVoltage=0  Measurements=None
      settings: SourceProductName=Simscape Electrical
  RfA : powerlib/Elements/Series RLC Branch  LConnTagsString=__new0  RConnTagsString=__new0  BranchType=R  Resistance=faultR  Inductance=1e-3  SetiL0=off  InitialCurrent=0  Capacitance=1e-6  Setx0=off  InitialVoltage=0  Measurements=None
      settings: SourceProductName=Simscape Electrical
  RfB : powerlib/Elements/Series RLC Branch  LConnTagsString=__new0  RConnTagsString=__new0  BranchType=R  Resistance=faultR  Inductance=1e-3  SetiL0=off  InitialCurrent=0  Capacitance=1e-6  Setx0=off  InitialVoltage=0  Measurements=None
      settings: SourceProductName=Simscape Electrical
  RfC : powerlib/Elements/Series RLC Branch  LConnTagsString=__new0  RConnTagsString=__new0  BranchType=R  Resistance=faultR  Inductance=1e-3  SetiL0=off  InitialCurrent=0  Capacitance=1e-6  Setx0=off  InitialVoltage=0  Measurements=None
      settings: SourceProductName=Simscape Electrical
  A : PMIOPort  Tag=PMCPort  Side=Left
  B : PMIOPort  Tag=PMCPort  Port=2  Side=Left
  C : PMIOPort  Tag=PMCPort  Port=3  Side=Left
  wires:
  faultA/1 -> &/1
  faultB/1 -> &1/1
  faultC/1 -> &2/1
  faultG/1 -> &3/1
  Tfault/1 -> &3/2, &2/2, &1/2, &/2
  &3/1 -> BreakerN/1
  &/1 -> BreakerA/1
  &1/1 -> BreakerB/1
  &2/1 -> BreakerC/1
  connections:
  B/RConn1 -- RB/LConn1 -- BreakerB/LConn1
  A/RConn1 -- BreakerA/LConn1 -- RA/LConn1
  RC/LConn1 -- C/RConn1 -- BreakerC/LConn1
  BreakerC/RConn1 -- RC/RConn1 -- RfC/LConn1
  RB/RConn1 -- RfB/LConn1 -- BreakerB/RConn1
  RA/RConn1 -- RfA/LConn1 -- BreakerA/RConn1
  BreakerN/LConn1 -- RN/LConn1 -- RfB/RConn1 -- RfA/RConn1 -- RfC/RConn1
  BreakerN/RConn1 -- Ground/LConn1 -- RN/RConn1

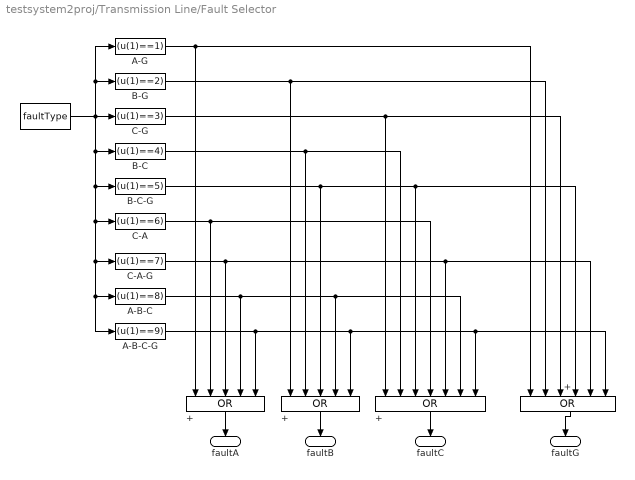
== system testsystem2proj/Transmission Line/Fault Selector ==
  " " : Constant  Value=faultType
  "  +" : Logic  Operator=OR  Inputs=7
  " +" : Logic  Operator=OR  Inputs=5
  + : Logic  Operator=OR  Inputs=5
  "+ " : Logic  Operator=OR  Inputs=6
  A-B-C : Fcn  Expr=(u(1)==8)
  A-B-C-G : Fcn  Expr=(u(1)==9)
  A-G : Fcn  Expr=(u(1)==1)
  B-C : Fcn  Expr=(u(1)==4)
  B-C-G : Fcn  Expr=(u(1)==5)
  B-G : Fcn  Expr=(u(1)==2)
  C-A : Fcn  Expr=(u(1)==6)
  C-A-G : Fcn  Expr=(u(1)==7)
  C-G : Fcn  Expr=(u(1)==3)
  faultA : Outport  InitialOutput=0
  faultB : Outport  Port=2  InitialOutput=0
  faultC : Outport  Port=3  InitialOutput=0
  faultG : Outport  Port=4  InitialOutput=0
  wires:
  " "/1 -> C-G/1, A-G/1, B-G/1, B-C/1, C-A/1, C-A-G/1, A-B-C/1, A-B-C-G/1, B-C-G/1
  +/1 -> faultA/1
  " +"/1 -> faultB/1
  "  +"/1 -> faultC/1
  "+ "/1 -> faultG/1
  A-G/1 -> "+ "/1, +/1
  C-A/1 -> "  +"/4, +/2
  B-G/1 -> " +"/1, "+ "/2
  B-C/1 -> "  +"/2, " +"/2
  B-C-G/1 -> "  +"/3, "+ "/4, " +"/3
  C-G/1 -> "  +"/1, "+ "/3
  C-A-G/1 -> "  +"/5, "+ "/5, +/3
  A-B-C-G/1 -> " +"/5, "  +"/7, "+ "/6, +/5
  A-B-C/1 -> " +"/4, "  +"/6, +/4

== system testsystem2proj/Protection Scheme/Backup Protection (Distance Protection)/DAB4 ==
  a : Inport
  AD & Buffer : S-Function  FunctionName=dab2  Parameters=winsize,fs,dx,resdis  SFunctionDeploymentMode=off  EnableBusSupport=off
  Analog Filter : TransferFcn  Numerator=num  Denominator=den
  Gain : Gain  Gain=G  SaturateOnIntegerOverflow=on  OutDataTypeStr=Inherit: Same as input  ParamDataTypeStr=Inherit: Same as input
  Zero-Order Hold : ZeroOrderHold  SampleTime=1/fs
  d : Outport  InitialOutput=[zeros(winsize,1)]
  wires:
  Analog Filter/1 -> Gain/1
  Gain/1 -> Zero-Order Hold/1
  Zero-Order Hold/1 -> AD & Buffer/1
  a/1 -> Analog Filter/1
  AD & Buffer/1 -> d/1

== system testsystem2proj/Protection Scheme/Backup Protection (Distance Protection)/DAB5 ==
  a : Inport
  AD & Buffer : S-Function  FunctionName=dab2  Parameters=winsize,fs,dx,resdis  SFunctionDeploymentMode=off  EnableBusSupport=off
  Analog Filter : TransferFcn  Numerator=num  Denominator=den
  Gain : Gain  Gain=G  SaturateOnIntegerOverflow=on  OutDataTypeStr=Inherit: Same as input  ParamDataTypeStr=Inherit: Same as input
  Zero-Order Hold : ZeroOrderHold  SampleTime=1/fs
  d : Outport  InitialOutput=[zeros(winsize,1)]
  wires:
  AD & Buffer/1 -> d/1
  a/1 -> Analog Filter/1
  Zero-Order Hold/1 -> AD & Buffer/1
  Gain/1 -> Zero-Order Hold/1
  Analog Filter/1 -> Gain/1

== system testsystem2proj/Protection Scheme/Backup Protection (Distance Protection)/DAB6 ==
  a : Inport
  AD & Buffer : S-Function  FunctionName=dab2  Parameters=winsize,fs,dx,resdis  SFunctionDeploymentMode=off  EnableBusSupport=off
  Analog Filter : TransferFcn  Numerator=num  Denominator=den
  Gain : Gain  Gain=G  SaturateOnIntegerOverflow=on  OutDataTypeStr=Inherit: Same as input  ParamDataTypeStr=Inherit: Same as input
  Zero-Order Hold : ZeroOrderHold  SampleTime=1/fs
  d : Outport  InitialOutput=[zeros(winsize,1)]
  wires:
  AD & Buffer/1 -> d/1
  a/1 -> Analog Filter/1
  Zero-Order Hold/1 -> AD & Buffer/1
  Gain/1 -> Zero-Order Hold/1
  Analog Filter/1 -> Gain/1

== system testsystem2proj/Protection Scheme/Backup Protection (Distance Protection)/DAB7 ==
  a : Inport
  AD & Buffer : S-Function  FunctionName=dab2  Parameters=winsize,fs,dx,resdis  SFunctionDeploymentMode=off  EnableBusSupport=off
  Analog Filter : TransferFcn  Numerator=num  Denominator=den
  Gain : Gain  Gain=G  SaturateOnIntegerOverflow=on  OutDataTypeStr=Inherit: Same as input  ParamDataTypeStr=Inherit: Same as input
  Zero-Order Hold : ZeroOrderHold  SampleTime=1/fs
  d : Outport  InitialOutput=[zeros(winsize,1)]
  wires:
  Analog Filter/1 -> Gain/1
  Gain/1 -> Zero-Order Hold/1
  Zero-Order Hold/1 -> AD & Buffer/1
  a/1 -> Analog Filter/1
  AD & Buffer/1 -> d/1

== system testsystem2proj/Protection Scheme/Backup Protection (Distance Protection)/DAB8 ==
  a : Inport
  AD & Buffer : S-Function  FunctionName=dab2  Parameters=winsize,fs,dx,resdis  SFunctionDeploymentMode=off  EnableBusSupport=off
  Analog Filter : TransferFcn  Numerator=num  Denominator=den
  Gain : Gain  Gain=G  SaturateOnIntegerOverflow=on  OutDataTypeStr=Inherit: Same as input  ParamDataTypeStr=Inherit: Same as input
  Zero-Order Hold : ZeroOrderHold  SampleTime=1/fs
  d : Outport  InitialOutput=[zeros(winsize,1)]
  wires:
  Analog Filter/1 -> Gain/1
  Gain/1 -> Zero-Order Hold/1
  Zero-Order Hold/1 -> AD & Buffer/1
  a/1 -> Analog Filter/1
  AD & Buffer/1 -> d/1

== system testsystem2proj/Protection Scheme/Backup Protection (Distance Protection)/DAB9 ==
  a : Inport
  AD & Buffer : S-Function  FunctionName=dab2  Parameters=winsize,fs,dx,resdis  SFunctionDeploymentMode=off  EnableBusSupport=off
  Analog Filter : TransferFcn  Numerator=num  Denominator=den
  Gain : Gain  Gain=G  SaturateOnIntegerOverflow=on  OutDataTypeStr=Inherit: Same as input  ParamDataTypeStr=Inherit: Same as input
  Zero-Order Hold : ZeroOrderHold  SampleTime=1/fs
  d : Outport  InitialOutput=[zeros(winsize,1)]
  wires:
  AD & Buffer/1 -> d/1
  a/1 -> Analog Filter/1
  Zero-Order Hold/1 -> AD & Buffer/1
  Gain/1 -> Zero-Order Hold/1
  Analog Filter/1 -> Gain/1

== system testsystem2proj/Protection Scheme/Backup Protection (Distance Protection)/Five-zone distance ==
  V: : Inport
  I: : Inport  Port=2
  BM : elements/BM  tpostv=none  plenv=4  tposti=none  pleni=4  tposts=none  plens=4  tpostz=none  plenz=4
  Mux3 : Mux  Inputs=3
  Terminator1 : Terminator
  ZC 1 : Subsystem  mask(Zone Comparator){typez=Free expression, z1=zone1, z2=zone2, z3=zone3, z4=zone4, zr=reversezone, fs=4*60}
      mask prompts: typez "shape"; z1 "Zone 1"; z2 "Zone 2"; z3 "Zone 3"; z4 "Zone 4"; zr "Reverse Zone"; fs "Sampling frecuency (Hz):"
      mask help: This block performs the zone comparison. Its inputs are the resistance and reactance signals. Four forward and one backward zones are implemented. The output that corresponds to the zone where the impedance is located is set to one while the rest of the outputs are zero Either the mho or free expression characteristics may be set. For the mho characteristic, the zones are defined by specifying the center of each circle (all the circles are tangent to the origin). For the free expression, arrays with consecutive vertices specify the polygons for each zone.
      mask init:
      | zc1;
      mask TypeOptions typez: Mho characteristic | Free expression
      mask Display:
      | plot(x1(:,1),x1(:,2));
      | plot(x2(:,1),x2(:,2));
      | plot(x3(:,1),x3(:,2));
      | plot(x4(:,1),x4(:,2));
      | plot(xr(:,1),xr(:,2));
  I : Outport
  II : Outport  Port=2
  III : Outport  Port=3
  IV : Outport  Port=4
  backward : Outport  Port=5
  wires:
  I:/1 -> BM/2
  V:/1 -> BM/1
  BM/4 -> ZC 1/1(Z)
  BM/1 -> Mux3/1
  BM/2 -> Mux3/2
  BM/3 -> Mux3/3
  ZC 1/1(1) -> I/1
  ZC 1/2(2) -> II/1
  ZC 1/3(3) -> III/1
  ZC 1/4(4) -> IV/1
  ZC 1/5(R) -> backward/1
  Mux3/1 -> Terminator1/1

== system testsystem2proj/Protection Scheme/Backup Protection (Distance Protection)/Five-zone distance1 ==
  V: : Inport
  I: : Inport  Port=2
  BM : elements/BM  tpostv=none  plenv=4  tposti=none  pleni=4  tposts=none  plens=4  tpostz=none  plenz=4
  Mux3 : Mux  Inputs=3
  Terminator : Terminator
  ZC 1 : Subsystem  mask(Zone Comparator){typez=Free expression, z1=zone1, z2=zone2, z3=zone3, z4=zone4, zr=reversezone, fs=4*60}
      mask prompts: typez "shape"; z1 "Zone 1"; z2 "Zone 2"; z3 "Zone 3"; z4 "Zone 4"; zr "Reverse Zone"; fs "Sampling frecuency (Hz):"
      mask help: This block performs the zone comparison. Its inputs are the resistance and reactance signals. Four forward and one backward zones are implemented. The output that corresponds to the zone where the impedance is located is set to one while the rest of the outputs are zero Either the mho or free expression characteristics may be set. For the mho characteristic, the zones are defined by specifying the center of each circle (all the circles are tangent to the origin). For the free expression, arrays with consecutive vertices specify the polygons for each zone.
      mask init:
      | zc1;
      mask TypeOptions typez: Mho characteristic | Free expression
      mask Display:
      | plot(x1(:,1),x1(:,2));
      | plot(x2(:,1),x2(:,2));
      | plot(x3(:,1),x3(:,2));
      | plot(x4(:,1),x4(:,2));
      | plot(xr(:,1),xr(:,2));
  I : Outport
  II : Outport  Port=2
  III : Outport  Port=3
  IV : Outport  Port=4
  backward : Outport  Port=5
  wires:
  ZC 1/5(R) -> backward/1
  ZC 1/4(4) -> IV/1
  ZC 1/3(3) -> III/1
  ZC 1/2(2) -> II/1
  ZC 1/1(1) -> I/1
  BM/3 -> Mux3/3
  BM/2 -> Mux3/2
  BM/1 -> Mux3/1
  BM/4 -> ZC 1/1(Z)
  V:/1 -> BM/1
  I:/1 -> BM/2
  Mux3/1 -> Terminator/1

== system testsystem2proj/Protection Scheme/Backup Protection (Distance Protection)/Five-zone distance2 ==
  V: : Inport
  I: : Inport  Port=2
  BM : elements/BM  tpostv=none  plenv=4  tposti=none  pleni=4  tposts=none  plens=4  tpostz=none  plenz=4
  Mux3 : Mux  Inputs=3
  Terminator : Terminator
  ZC 1 : Subsystem  mask(Zone Comparator){typez=Free expression, z1=zone1, z2=zone2, z3=zone3, z4=zone4, zr=reversezone, fs=4*60}
      mask prompts: typez "shape"; z1 "Zone 1"; z2 "Zone 2"; z3 "Zone 3"; z4 "Zone 4"; zr "Reverse Zone"; fs "Sampling frecuency (Hz):"
      mask help: This block performs the zone comparison. Its inputs are the resistance and reactance signals. Four forward and one backward zones are implemented. The output that corresponds to the zone where the impedance is located is set to one while the rest of the outputs are zero Either the mho or free expression characteristics may be set. For the mho characteristic, the zones are defined by specifying the center of each circle (all the circles are tangent to the origin). For the free expression, arrays with consecutive vertices specify the polygons for each zone.
      mask init:
      | zc1;
      mask TypeOptions typez: Mho characteristic | Free expression
      mask Display:
      | plot(x1(:,1),x1(:,2));
      | plot(x2(:,1),x2(:,2));
      | plot(x3(:,1),x3(:,2));
      | plot(x4(:,1),x4(:,2));
      | plot(xr(:,1),xr(:,2));
  I : Outport
  II : Outport  Port=2
  III : Outport  Port=3
  IV : Outport  Port=4
  backward : Outport  Port=5
  wires:
  I:/1 -> BM/2
  V:/1 -> BM/1
  BM/4 -> ZC 1/1(Z)
  BM/1 -> Mux3/1
  BM/2 -> Mux3/2
  BM/3 -> Mux3/3
  ZC 1/1(1) -> I/1
  ZC 1/2(2) -> II/1
  ZC 1/3(3) -> III/1
  ZC 1/4(4) -> IV/1
  ZC 1/5(R) -> backward/1
  Mux3/1 -> Terminator/1
